simulink model "PubIfDecisionVSM_HOD"  (R2020b)
settings: Solver=FixedStepDiscrete  StartTime=0.0  StopTime=Inf  RelTol=1e-3
PostLoadFcn:
  | if any(exist('dsrtsu_mdlpostloadfcn', 'file') ~= 0), dsrtsu_mdlpostloadfcn('Execute', bdroot); end
InitFcn:
  | , if any(exist('dsmpb_private', 'file') ~= 0), dsmpb_private('dsmpb_mdlclblib', 'Init', bdroot); end,
PreSaveFcn:
  | , if any(exist('dsmpb_private', 'file') ~= 0), dsmpb_private('dsmpb_mdlclblib', 'PreSave', bdroot); end,
CloseFcn:
  | , if any(exist('dsmpb_private', 'file') ~= 0), dsmpb_private('dsmpb_mdlclblib', 'Close', bdroot); end,
settings Model: DataDictionary=enumsss.sldd  RTICANMMDATA=struct('GeneralSetupData',struct('modelroot','C:\Users\GW00133806\Desktop\ADAS_Store\Adas\VSM\HOD','generalsettings',struct('filesettings',struct('destfolder',struct('Name','RTICANMM_FILES','Check',1),'buildfolder',struct('Name','.','Check',1),'AbsDestfolder',struct('Name','C:\Users\GW00133806\Desktop\ADAS_Store\Adas\VSM\HOD\RTICANMM_FILES'),'AbsBuildfolder',struct('Name','C:\Users\GW00133806\Desktop\ADAS_Store\Adas\VSM\HOD'))),'options',struct('addpaths',1,'rmpaths',1,'addtrcexclusion',false,'cannavigator',struct('checkmonitoring',0),'show_usrtrc',0,'use_usrtrc',0),'advanced',struct('options',ones(1,100)),'MPSetup',{{}},'RTI',struct('Type','DSRT','Ver','4.2','Date','02-Nov-2019'),'modelname','PubIfDecisionVSM_HOD','block','PubIfDecisionVSM_HOD'))  DSRTSU_INTERNAL_RTIFPGA=150  Creator=GW00166368  LastModifiedBy=GW00201299
settings OptimizationCC: BlockReduction=off  ConditionallyExecuteInputs=off  OptimizeBlockIOStorage=off  BufferReuse=off
settings DebuggingCC: TasksWithSamePriorityMsg=none  UnderSpecifiedDimensionMsg=warning
settings HardwareCC: ProdBitPerPointer=32  ProdBitPerSizeT=32  ProdBitPerPtrDiffT=32  ProdLargestAtomicInteger=Integer  ProdWordSize=32  ProdHWDeviceType=Custom Processor->Custom
settings ModelReferenceCC: EnableParallelModelReferenceBuilds=on  ModelReferenceNumInstancesAllowed=Single
settings SFSimCC: MATLABDynamicMemAlloc=off
settings RTWCC: Description=dSPACE Run-Time Target (for VEOS on Windows and ConfigurationDesk)  SystemTargetFile=dsrt.tlc  GenCodeOnly=on  MakeCommand=make_dsrt  TemplateMakefile=dsrt_default_tmf  RTWVerbose=off
settings CodeAppCC: MaxIdLength=128
settings STFCustomTargetCC: TargetLangStandard=C99 (ISO)  ParMdlRefBuildCompliant=on  ConcurrentExecutionCompliant=off  CPPClassGenCompliant=off  GRTInterface=off  SystemTargetFile=dsrt.tlc
settings GRTTargetCC: CompOptLevelCompliant=off  ConcurrentExecutionCompliant=off  CombineOutputUpdateFcns=off  MatFileLogging=off  CPPClassGenCompliant=off  UseToolchainInfoCompliant=off

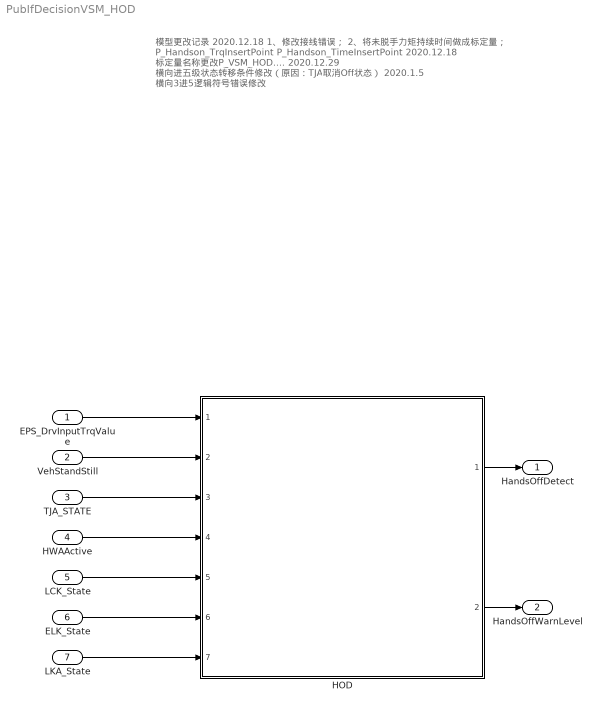
== system PubIfDecisionVSM_HOD ==
  note: 模型更改记录
      | 2020.12.18
      | 1、修改接线错误；
      | 2、将未脱手力矩持续时间做成标定量；
      |      P_Handson_TrqInsertPoint
      |      P_Handson_TimeInsertPoint
      | 2020.12.18
      | 标定量名称更改P_VSM_HOD....
      | 2020.12.29
      | 横向进五级状态转移条件修改（原因：TJA取消Off状态）
      | 2020.1.5
      | 横向3进5逻辑符号错误修改
  EPS_DrvInputTrqValue : Inport  OutDataTypeStr=single
  VehStandStill : Inport  Port=2  OutDataTypeStr=uint8
  TJA_STATE : Inport  Port=3  OutDataTypeStr=Enum: TJA_STATE
  HWAActive : Inport  Port=4  OutDataTypeStr=boolean
  LCK_State : Inport  Port=5  OutDataTypeStr=Enum: LCK_STATE
  ELK_State : Inport  Port=6  OutDataTypeStr=Enum: ELKSTATE
  LKA_State : Inport  Port=7  OutDataTypeStr=Enum: STATE
  HOD : Subsystem  ReferencedSubsystem=PvtSubSys_VSM_HOD
  HandsOffDetect : Outport  OutDataTypeStr=boolean
  HandsOffWarnLevel : Outport  Port=2  OutDataTypeStr=uint8
  wires:
  LCK_State/1 -> HOD/5
  EPS_DrvInputTrqValue/1 -> HOD/1
  HOD/1 -> HandsOffDetect/1
  HOD/2 -> HandsOffWarnLevel/1
  ELK_State/1 -> HOD/6
  VehStandStill/1 -> HOD/2
  HWAActive/1 -> HOD/4
  LKA_State/1 -> HOD/7
  TJA_STATE/1 -> HOD/3
